simulink model "ekf_arduino"  (R2015a)
settings: Solver=ode3  StartTime=0.0  StopTime=10.0  FixedStep=1/200  RelTol=1e-3
libraries: PoliArd x6
settings Model: ExtModeTrigDuration=2  Creator=User  LastModifiedBy=gianl
settings OptimizationCC: OptimizeModelRefInitCode=on  LifeSpan=1
settings DebuggingCC: UnderspecifiedInitializationDetection=Classic  MergeDetectMultiDrivingBlocksExec=none
settings HardwareCC: ProdLargestAtomicInteger=Long  ProdLargestAtomicFloat=Double  ProdEndianess=LittleEndian  ProdHWDeviceType=ARM Compatible->ARM Cortex
settings RTWCC: SystemTargetFile=realtime.tlc  GenerateMakefile=off  TemplateMakefile=realtime.tmf  Description=Run on Target Hardware  RTWVerbose=off
settings ERTTargetCC: CombineOutputUpdateFcns=off  ExtModeTransport=3  ExtModeMexFile=ext_serial_win32_comm_rtt  ExtModeMexArgs=0 1 9600  InlinedParameterPlacement=Hierarchical  ERTSrcFileBannerTemplate=realtime_code_template.cgt  ERTHdrFileBannerTemplate=realtime_code_template.cgt  ERTDataSrcFileTemplate=realtime_code_template.cgt  ERTDataHdrFileTemplate=realtime_code_template.cgt  ERTCustomFileTemplate=realtime_file_process.tlc

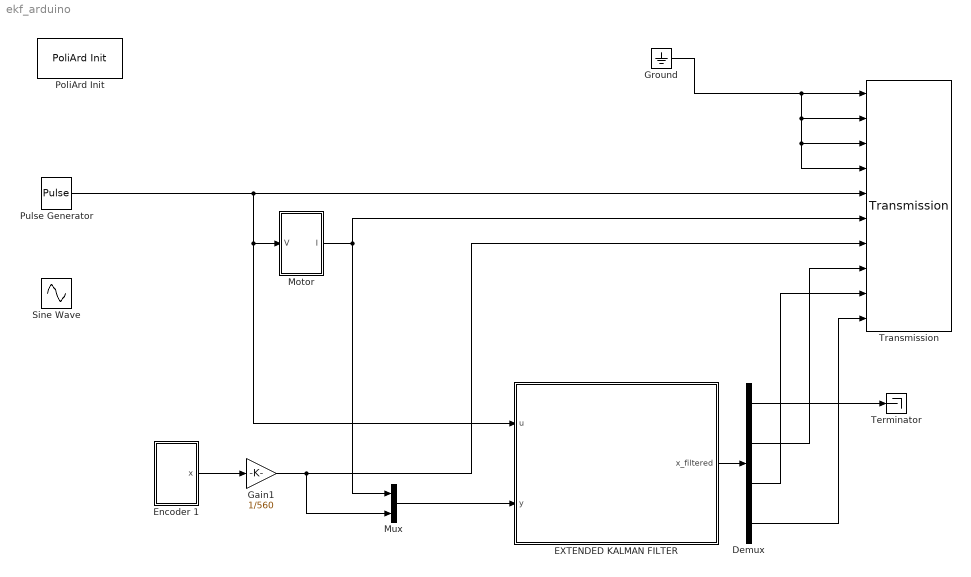
== system ekf_arduino ==
  Demux : Demux
  EXTENDED KALMAN FILTER : MATLAB Function  TreatAsAtomicUnit=on
      settings: PermitHierarchicalResolution=ParametersOnly
  Encoder 1 : Subsystem
  Gain1 : Gain  Gain=1/560
  Ground : Ground
  Motor : Subsystem
  Mux : Mux  Inputs=2
  PoliArd Init : PoliArd/PoliArd Init
  Pulse Generator : DiscretePulseGenerator  PulseType=Time based  Period=10  PulseWidth=5
  Sine Wave : Sin  Frequency=2*pi  SampleTime=0
  Terminator : Terminator
  Transmission : PoliArd/Transmission  sample_freq=200  sig_to_send=6
  wires:
  Ground/1 -> Transmission/1, Transmission/2, Transmission/4, Transmission/3
  Mux/1 -> EXTENDED KALMAN FILTER/2(y)
  EXTENDED KALMAN FILTER/1(x_filtered) -> Demux/1
  Demux/2 -> Transmission/8
  Demux/1 -> Terminator/1
  Demux/3 -> Transmission/9
  Demux/4 -> Transmission/10
  Pulse Generator/1 -> EXTENDED KALMAN FILTER/1(u), Motor/1(V), Transmission/5
  Motor/1(I) -> Transmission/6, Mux/1
  Gain1/1 -> Mux/2, Transmission/7
  Encoder 1/1(x) -> Gain1/1

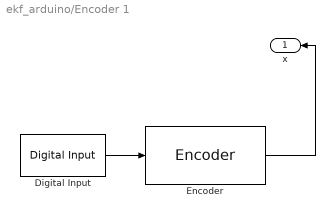
== system ekf_arduino/Encoder 1 ==
  Digital Input : PoliArd/Digital Input  DI_pin=2  DIsample=1/200
  Encoder : PoliArd/Encoder  EncoderID=3  dt_enc=-1
  x : Outport
  wires:
  Digital Input/1 -> Encoder/1
  Encoder/1 -> x/1

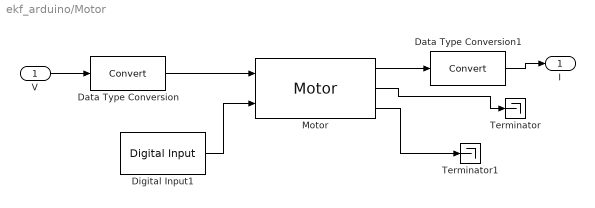
== system ekf_arduino/Motor ==
  V : Inport
  Data Type Conversion : DataTypeConversion
  Data Type Conversion1 : DataTypeConversion
  Digital Input1 : PoliArd/Digital Input  DI_pin=3  DIsample=1/200
  Motor : PoliArd/Motor  MotorID=2  DC_bus_mask=12  dt_mot=1/200
  Terminator : Terminator
  Terminator1 : Terminator
  I : Outport
  wires:
  Data Type Conversion/1 -> Motor/1
  Digital Input1/1 -> Motor/2
  V/1 -> Data Type Conversion/1
  Motor/3 -> Terminator1/1
  Motor/2 -> Terminator/1
  Motor/1 -> Data Type Conversion1/1
  Data Type Conversion1/1 -> I/1

== matlab function ekf_arduino/EXTENDED KALMAN FILTER ==
  data: u input; y input; x_filtered output
function x_filtered  = ekf(u, y)
    %% Discrete Kalman filter for continous system
    % Inputs:
    % u: input to the system
    % y: output of the system
    % Output:
    % x_filtered: Kalman state estimate
    
    
    % P and xhat need to be updated each iteration
    % The other variables are parameters of the real vector.
    persistent P xhat Q R Res L M Gamma C B H
    
    if isempty(P)%First iteration, initialize values
        P = eye(4);
        xhat = [0; 0; 0; 100];
        Q = 1e-10*eye(4);
        R = diag([0.0127; 1e-10]);
        
        M = 1.8;
%         C = 8.9973; %low
        C = 9.5558;
        Res = 1.3;
        L = 0.0024;
        Gamma = -2.068;
        
        B = 1/200.*[1/L; 0; 0; 0]; %Discretized Input Matrix B
        H = [1 0 0 0; 0 100 0 0]; % Output current and position
    end
    
    % Linearize the continuos system around xhat
    A = [ -Res/L,       0,              0,      0; ...
          0,            0,              1,      0; ...
        Gamma/M,        -xhat(4)/M,     -C/M,   -xhat(2)/M; ...
        0,              0,              0,      0];
    
    A = eye(4) + 1/200.*A; %Discretize A

    % Real nonlinear system computed in xhat
    f = [ -Res/L*xhat(1); ...
          xhat(3); ...
          Gamma/M*xhat(1) - xhat(4)*xhat(2)/M - C/M*xhat(3); ...
          0 ];
     
    % Discretize f 
    f = 1/200.*f;
    f = f + xhat;
    
    % Update Prediction
    x_pred = f + B*u;   % x_k+1 = f(x_k) + Bu_k
    y_pred = H*x_pred;  % y_k+1 = H*x_k+1
    
    % Update P
    P = A*P*A' + Q;
    
    % Update Kalman Gain
    K = P*H'/(H*P*H'+R);
    
    %Update Prediction
    xhat = x_pred + K*(y - y_pred);
    
    % Update P
    P = (eye(size(K*H)) - K*H)*P;
    
    % Output the state-estimate
    x_filtered = xhat;
